simulink model "parallel_decimation_testbench_4inputs"  (Simulink 7.4)
settings: Solver=ode45  StartTime=0.0  StopTime=100  RelTol=1e-3
libraries: xbsIndex_r4 x25, simulink x2
settings Model: Creator=chenhong  LastModifiedBy=chenhong

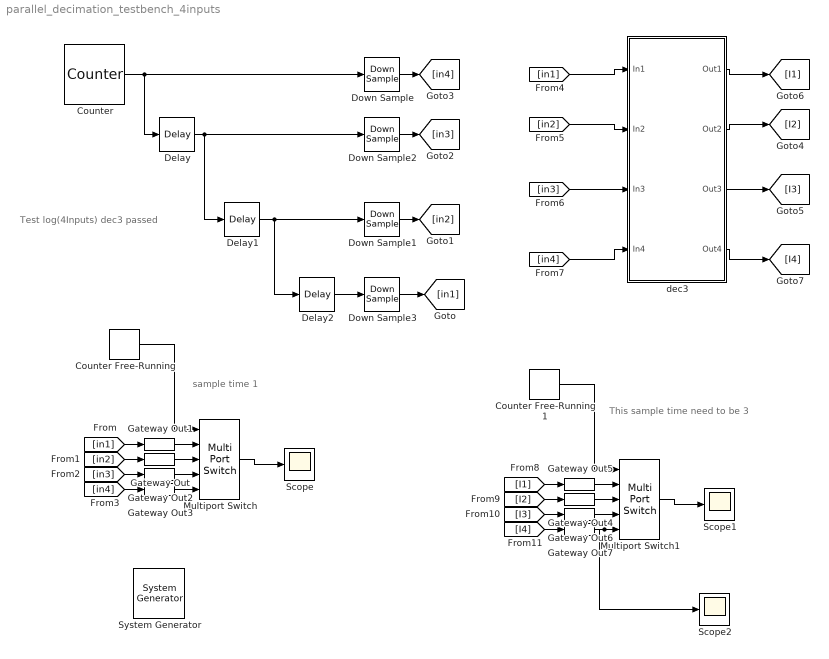
== system parallel_decimation_testbench_4inputs ==
  note: This sample time need to be 3
  note: sample time 1
  note: Test log(4Inputs)
      | dec3 passed
  " System Generator" : xbsIndex_r4/ System Generator  Tag=genX  SystemSampleTime=-1  xilinxfamily=Virtex6  part=xc6vsx315t  speed=-3  package=ff1156  synthesis_tool=XST  clock_wrapper=Clock Enables  directory=./netlist  testbench=off  simulink_period=1  sysclk_period=10  dcm_input_clock_period=10  incr_netlist=off  trim_vbits=Everywhere in SubSystem  dbl_ovrd=According to Block Masks  core_generation=According to Block Masks  run_coregen=off  deprecated_control=off  eval_field=0  block_type=sysgen
      settings: block_version=11.4
  Counter : xbsIndex_r4/Counter  cnt_type=Free Running  cnt_to=Inf  operation=Up  start_count=0  cnt_by_val=1  arith_type=Unsigned  n_bits=8  bin_pt=0  load_pin=off  rst=off  en=off  explicit_period=on  period=1  dbl_ovrd=off  use_behavioral_HDL=off  implementation=Fabric  block_type=counter
      settings: block_version=11.4
  Counter Free-Running : simulink/Sources/Counter Free-Running  SystemSampleTime=-1  NumBits=2  tsamp=1
  Counter Free-Running1 : simulink/Sources/Counter Free-Running  SystemSampleTime=-1  NumBits=2  tsamp=3
  Delay : xbsIndex_r4/Delay  en=off  latency=1  dbl_ovrd=off  reg_retiming=off  block_type=delay
      settings: block_version=11.4
  Delay1 : xbsIndex_r4/Delay  en=off  latency=1  dbl_ovrd=off  reg_retiming=off  block_type=delay
      settings: block_version=11.4
  Delay2 : xbsIndex_r4/Delay  en=off  latency=1  dbl_ovrd=off  reg_retiming=off  block_type=delay
      settings: block_version=11.4
  Down Sample{,1..3} (4 alike) : xbsIndex_r4/Down Sample  sample_ratio=4  sample_phase="Last Value of Frame  (most efficient)"  en=off  latency=1  dbl_ovrd=off  block_type=dsamp
      settings: block_version=11.4
  Gateway Out{,1..7} (8 alike) : xbsIndex_r4/Gateway Out  hdl_port=off  timing_constraint=None  locs_specified=off  LOCs={}  block_type=gatewayout
      settings: infoedit="Gateway out block.  Converts Xilinx fixed point inputs into ouputs of type Simulink integer, double, or fixed point.<br><br>Hardware notes:  In hardware these blocks become top level output ports or are discarded, depending on how they are configured."  block_version=11.4
  Multiport Switch : MultiPortSwitch  Inputs=4  zeroidx=on  OutDataType=fixdt(1, 16)  OutScaling=2^0  SampleTime=1
  Multiport Switch1 : MultiPortSwitch  Inputs=4  zeroidx=on  OutDataType=fixdt(1, 16)  OutScaling=2^0  SampleTime=3
  Scope : Scope
  Scope1 : Scope
  Scope2 : Scope
      settings: SaveName=ScopeData2
  dec3 : Subsystem
  wires:
  Counter/1 -> Down Sample/1, Delay/1
  Delay/1 -> Down Sample2/1, Delay1/1
  Delay1/1 -> Down Sample1/1, Delay2/1
  Delay2/1 -> Down Sample3/1
  Counter Free-Running/1 -> Multiport Switch/1
  Down Sample/1 -> [in4]
  Down Sample2/1 -> [in3]
  Down Sample1/1 -> [in2]
  Down Sample3/1 -> [in1]
  [in1] -> Gateway Out1/1
  [in2] -> Gateway Out/1
  [in3] -> Gateway Out2/1
  [in4] -> Gateway Out3/1
  Gateway Out1/1 -> Multiport Switch/2
  Gateway Out/1 -> Multiport Switch/3
  Gateway Out2/1 -> Multiport Switch/4
  Gateway Out3/1 -> Multiport Switch/5
  Multiport Switch/1 -> Scope/1
  [in2] -> dec3/2(In2)
  [in3] -> dec3/3(In3)
  [in1] -> dec3/1(In1)
  [in4] -> dec3/4(In4)
  dec3/2(Out2) -> [I2]
  dec3/3(Out3) -> [I3]
  dec3/1(Out1) -> [I1]
  dec3/4(Out4) -> [I4]
  Counter Free-Running1/1 -> Multiport Switch1/1
  [I1] -> Gateway Out5/1
  [I2] -> Gateway Out4/1
  [I3] -> Gateway Out6/1
  [I4] -> Gateway Out7/1
  Gateway Out5/1 -> Multiport Switch1/2
  Gateway Out4/1 -> Multiport Switch1/3
  Gateway Out6/1 -> Multiport Switch1/4
  Gateway Out7/1 -> Multiport Switch1/5, Scope2/1
  Multiport Switch1/1 -> Scope1/1

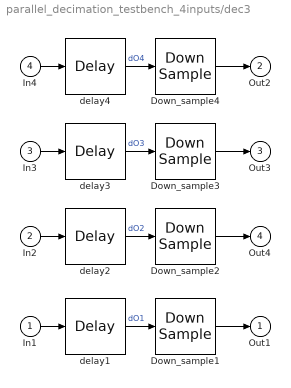
== system parallel_decimation_testbench_4inputs/dec3 ==
  In1 : Inport
  In2 : Inport  Port=2
  In3 : Inport  Port=3
  In4 : Inport  Port=4
  Down_sample{1..4} (4 alike) : xbsIndex_r4/Down Sample  sample_ratio=3  sample_phase="Last Value of Frame  (most efficient)"  en=off  latency=1  dbl_ovrd=off  block_type=dsamp
      settings: block_version=11.4
  delay1 : xbsIndex_r4/Delay  en=off  latency=2  dbl_ovrd=off  reg_retiming=off  block_type=delay
      settings: block_version=11.4
  delay2 : xbsIndex_r4/Delay  en=off  latency=0  dbl_ovrd=off  reg_retiming=off  block_type=delay
      settings: block_version=11.4
  delay3 : xbsIndex_r4/Delay  en=off  latency=1  dbl_ovrd=off  reg_retiming=off  block_type=delay
      settings: block_version=11.4
  delay4 : xbsIndex_r4/Delay  en=off  latency=2  dbl_ovrd=off  reg_retiming=off  block_type=delay
      settings: block_version=11.4
  Out1 : Outport
  Out2 : Outport  Port=2
  Out3 : Outport  Port=3
  Out4 : Outport  Port=4
  wires:
  delay4/1 -> Down_sample4/1  "dO4"
  In4/1 -> delay4/1
  Down_sample3/1 -> Out3/1
  delay2/1 -> Down_sample2/1  "dO2"
  In2/1 -> delay2/1
  Down_sample1/1 -> Out1/1
  In1/1 -> delay1/1
  delay1/1 -> Down_sample1/1  "dO1"
  Down_sample2/1 -> Out4/1
  In3/1 -> delay3/1
  delay3/1 -> Down_sample3/1  "dO3"
  Down_sample4/1 -> Out2/1
